simulink model "Ieee14_CC"  (R2023b)
settings: Solver=ode1  StartTime=0.0  StopTime=3600  FixedStep=1e-3  MaxStep=1e-4  RelTol=1e-3
model workspace (MAT data in the model file):
  pruebaValor = 0
libraries: dspnetwork x116, spsThreePhaseVIMeasurementLib x39, spsThreePhaseBreakerLib x21, spsLoadFlowBusLib x19, spsThreePhaseSeriesRLCBranchLib x16, spsThreePhaseFaultLib x16, source_mod x14, spsThreePhaseTransformerTwoWindingsLib x4, spsThreePhaseSourceLib x2, simulink x1, spspowerguiLib x1
(part 2 of 3)

== system Ieee14_CC/CB 0 ==
  Terminator : Terminator
  Three-Phase Breaker3 : spsThreePhaseBreakerLib/Three-Phase Breaker  InitialState=closed  SwitchA=on  SwitchB=on  SwitchC=on  SwitchTimes=[0.2]  External=on  BreakerResistance=0.01  SnubberResistance=1e6  SnubberCapacitance=inf  Measurements=Breaker voltages and currents
  UDP Receive : dspnetwork/UDP Receive  localURL='0.0.0.0'  localPort=30000  remoteURL='0.0.0.0'  remotePort=-1  recvBufferSize=2  dims=1  signalDatatype=uint16  isComplex=off  isVarSize=off  showBlockingTime=on  blockingTime=0  sampletime=0.1  blockPlatform=LINUX
  a : PMIOPort  Side=Left
  b : PMIOPort  Port=2  Side=Left
  c : PMIOPort  Port=3  Side=Left
  A : PMIOPort  Port=4  Side=Right
  B : PMIOPort  Port=5  Side=Right
  C : PMIOPort  Port=6  Side=Right
  com : Outport
  wires:
  UDP Receive/1 -> Three-Phase Breaker3/1, com/1
  UDP Receive/2 -> Terminator/1
  connections:
  b/RConn1 -- Three-Phase Breaker3/RConn2
  c/RConn1 -- Three-Phase Breaker3/RConn3
  A/RConn1 -- Three-Phase Breaker3/LConn1
  Three-Phase Breaker3/LConn2 -- B/RConn1
  C/RConn1 -- Three-Phase Breaker3/LConn3
  a/RConn1 -- Three-Phase Breaker3/RConn1

== system Ieee14_CC/CB 1 ==
  Terminator : Terminator
  Three-Phase Breaker3 : spsThreePhaseBreakerLib/Three-Phase Breaker  InitialState=closed  SwitchA=on  SwitchB=on  SwitchC=on  SwitchTimes=[0.2]  External=on  BreakerResistance=0.01  SnubberResistance=1e6  SnubberCapacitance=inf  Measurements=Breaker voltages and currents
  UDP Receive : dspnetwork/UDP Receive  localURL='0.0.0.0'  localPort=30001  remoteURL='0.0.0.0'  remotePort=-1  recvBufferSize=2  dims=1  signalDatatype=uint16  isComplex=off  isVarSize=off  showBlockingTime=on  blockingTime=0  sampletime=0.1  blockPlatform=LINUX
  a : PMIOPort  Side=Left
  b : PMIOPort  Port=2  Side=Left
  c : PMIOPort  Port=3  Side=Left
  A : PMIOPort  Port=4  Side=Right
  B : PMIOPort  Port=5  Side=Right
  C : PMIOPort  Port=6  Side=Right
  com : Outport
  wires:
  UDP Receive/1 -> Three-Phase Breaker3/1, com/1
  UDP Receive/2 -> Terminator/1
  connections:
  b/RConn1 -- Three-Phase Breaker3/RConn2
  c/RConn1 -- Three-Phase Breaker3/RConn3
  A/RConn1 -- Three-Phase Breaker3/LConn1
  Three-Phase Breaker3/LConn2 -- B/RConn1
  C/RConn1 -- Three-Phase Breaker3/LConn3
  a/RConn1 -- Three-Phase Breaker3/RConn1

== system Ieee14_CC/CB 10 ==
  Terminator : Terminator
  Three-Phase Breaker3 : spsThreePhaseBreakerLib/Three-Phase Breaker  InitialState=closed  SwitchA=on  SwitchB=on  SwitchC=on  SwitchTimes=[0.2]  External=on  BreakerResistance=0.01  SnubberResistance=1e6  SnubberCapacitance=inf  Measurements=Breaker voltages and currents
  UDP Receive : dspnetwork/UDP Receive  localURL='0.0.0.0'  localPort=30010  remoteURL='0.0.0.0'  remotePort=-1  recvBufferSize=2  dims=1  signalDatatype=uint16  isComplex=off  isVarSize=off  showBlockingTime=on  blockingTime=0  sampletime=0.1  blockPlatform=LINUX
  a : PMIOPort  Side=Left
  b : PMIOPort  Port=2  Side=Left
  c : PMIOPort  Port=3  Side=Left
  A : PMIOPort  Port=4  Side=Right
  B : PMIOPort  Port=5  Side=Right
  C : PMIOPort  Port=6  Side=Right
  com : Outport
  wires:
  UDP Receive/1 -> Three-Phase Breaker3/1, com/1
  UDP Receive/2 -> Terminator/1
  connections:
  b/RConn1 -- Three-Phase Breaker3/RConn2
  c/RConn1 -- Three-Phase Breaker3/RConn3
  A/RConn1 -- Three-Phase Breaker3/LConn1
  Three-Phase Breaker3/LConn2 -- B/RConn1
  C/RConn1 -- Three-Phase Breaker3/LConn3
  a/RConn1 -- Three-Phase Breaker3/RConn1

== system Ieee14_CC/CB 11 ==
  Terminator : Terminator
  Three-Phase Breaker3 : spsThreePhaseBreakerLib/Three-Phase Breaker  InitialState=closed  SwitchA=on  SwitchB=on  SwitchC=on  SwitchTimes=[0.2]  External=on  BreakerResistance=0.01  SnubberResistance=1e6  SnubberCapacitance=inf  Measurements=Breaker voltages and currents
  UDP Receive : dspnetwork/UDP Receive  localURL='0.0.0.0'  localPort=30011  remoteURL='0.0.0.0'  remotePort=-1  recvBufferSize=2  dims=1  signalDatatype=uint16  isComplex=off  isVarSize=off  showBlockingTime=on  blockingTime=0  sampletime=0.1  blockPlatform=LINUX
  a : PMIOPort  Side=Left
  b : PMIOPort  Port=2  Side=Left
  c : PMIOPort  Port=3  Side=Left
  A : PMIOPort  Port=4  Side=Right
  B : PMIOPort  Port=5  Side=Right
  C : PMIOPort  Port=6  Side=Right
  com : Outport
  wires:
  UDP Receive/1 -> Three-Phase Breaker3/1, com/1
  UDP Receive/2 -> Terminator/1
  connections:
  b/RConn1 -- Three-Phase Breaker3/RConn2
  c/RConn1 -- Three-Phase Breaker3/RConn3
  A/RConn1 -- Three-Phase Breaker3/LConn1
  Three-Phase Breaker3/LConn2 -- B/RConn1
  C/RConn1 -- Three-Phase Breaker3/LConn3
  a/RConn1 -- Three-Phase Breaker3/RConn1

== system Ieee14_CC/CB 12 ==
  Terminator : Terminator
  Three-Phase Breaker3 : spsThreePhaseBreakerLib/Three-Phase Breaker  InitialState=closed  SwitchA=on  SwitchB=on  SwitchC=on  SwitchTimes=[0.2]  External=on  BreakerResistance=0.01  SnubberResistance=1e6  SnubberCapacitance=inf  Measurements=Breaker voltages and currents
  UDP Receive : dspnetwork/UDP Receive  localURL='0.0.0.0'  localPort=30012  remoteURL='0.0.0.0'  remotePort=-1  recvBufferSize=2  dims=1  signalDatatype=uint16  isComplex=off  isVarSize=off  showBlockingTime=on  blockingTime=0  sampletime=0.1  blockPlatform=LINUX
  a : PMIOPort  Side=Left
  b : PMIOPort  Port=2  Side=Left
  c : PMIOPort  Port=3  Side=Left
  A : PMIOPort  Port=4  Side=Right
  B : PMIOPort  Port=5  Side=Right
  C : PMIOPort  Port=6  Side=Right
  com : Outport
  wires:
  UDP Receive/1 -> Three-Phase Breaker3/1, com/1
  UDP Receive/2 -> Terminator/1
  connections:
  b/RConn1 -- Three-Phase Breaker3/RConn2
  c/RConn1 -- Three-Phase Breaker3/RConn3
  A/RConn1 -- Three-Phase Breaker3/LConn1
  Three-Phase Breaker3/LConn2 -- B/RConn1
  C/RConn1 -- Three-Phase Breaker3/LConn3
  a/RConn1 -- Three-Phase Breaker3/RConn1

== system Ieee14_CC/CB 13 ==
  Terminator : Terminator
  Three-Phase Breaker3 : spsThreePhaseBreakerLib/Three-Phase Breaker  InitialState=closed  SwitchA=on  SwitchB=on  SwitchC=on  SwitchTimes=[0.2]  External=on  BreakerResistance=0.01  SnubberResistance=1e6  SnubberCapacitance=inf  Measurements=Breaker voltages and currents
  UDP Receive : dspnetwork/UDP Receive  localURL='0.0.0.0'  localPort=30013  remoteURL='0.0.0.0'  remotePort=-1  recvBufferSize=2  dims=1  signalDatatype=uint16  isComplex=off  isVarSize=off  showBlockingTime=on  blockingTime=0  sampletime=0.1  blockPlatform=LINUX
  a : PMIOPort  Side=Left
  b : PMIOPort  Port=2  Side=Left
  c : PMIOPort  Port=3  Side=Left
  A : PMIOPort  Port=4  Side=Right
  B : PMIOPort  Port=5  Side=Right
  C : PMIOPort  Port=6  Side=Right
  com : Outport
  wires:
  UDP Receive/1 -> Three-Phase Breaker3/1, com/1
  UDP Receive/2 -> Terminator/1
  connections:
  b/RConn1 -- Three-Phase Breaker3/RConn2
  c/RConn1 -- Three-Phase Breaker3/RConn3
  A/RConn1 -- Three-Phase Breaker3/LConn1
  Three-Phase Breaker3/LConn2 -- B/RConn1
  C/RConn1 -- Three-Phase Breaker3/LConn3
  a/RConn1 -- Three-Phase Breaker3/RConn1

== system Ieee14_CC/CB 14 ==
  Terminator : Terminator
  Three-Phase Breaker3 : spsThreePhaseBreakerLib/Three-Phase Breaker  InitialState=closed  SwitchA=on  SwitchB=on  SwitchC=on  SwitchTimes=[0.2]  External=on  BreakerResistance=0.01  SnubberResistance=1e6  SnubberCapacitance=inf  Measurements=Breaker voltages and currents
  UDP Receive : dspnetwork/UDP Receive  localURL='0.0.0.0'  localPort=30014  remoteURL='0.0.0.0'  remotePort=-1  recvBufferSize=2  dims=1  signalDatatype=uint16  isComplex=off  isVarSize=off  showBlockingTime=on  blockingTime=0  sampletime=0.1  blockPlatform=LINUX
  a : PMIOPort  Side=Left
  b : PMIOPort  Port=2  Side=Left
  c : PMIOPort  Port=3  Side=Left
  A : PMIOPort  Port=4  Side=Right
  B : PMIOPort  Port=5  Side=Right
  C : PMIOPort  Port=6  Side=Right
  com : Outport
  wires:
  UDP Receive/1 -> Three-Phase Breaker3/1, com/1
  UDP Receive/2 -> Terminator/1
  connections:
  b/RConn1 -- Three-Phase Breaker3/RConn2
  c/RConn1 -- Three-Phase Breaker3/RConn3
  A/RConn1 -- Three-Phase Breaker3/LConn1
  Three-Phase Breaker3/LConn2 -- B/RConn1
  C/RConn1 -- Three-Phase Breaker3/LConn3
  a/RConn1 -- Three-Phase Breaker3/RConn1

== system Ieee14_CC/CB 15 ==
  Terminator : Terminator
  Three-Phase Breaker3 : spsThreePhaseBreakerLib/Three-Phase Breaker  InitialState=closed  SwitchA=on  SwitchB=on  SwitchC=on  SwitchTimes=[0.2]  External=on  BreakerResistance=0.01  SnubberResistance=1e6  SnubberCapacitance=inf  Measurements=Breaker voltages and currents
  UDP Receive : dspnetwork/UDP Receive  localURL='0.0.0.0'  localPort=30015  remoteURL='0.0.0.0'  remotePort=-1  recvBufferSize=2  dims=1  signalDatatype=uint16  isComplex=off  isVarSize=off  showBlockingTime=on  blockingTime=0  sampletime=0.1  blockPlatform=LINUX
  a : PMIOPort  Side=Left
  b : PMIOPort  Port=2  Side=Left
  c : PMIOPort  Port=3  Side=Left
  A : PMIOPort  Port=4  Side=Right
  B : PMIOPort  Port=5  Side=Right
  C : PMIOPort  Port=6  Side=Right
  com : Outport
  wires:
  UDP Receive/1 -> Three-Phase Breaker3/1, com/1
  UDP Receive/2 -> Terminator/1
  connections:
  b/RConn1 -- Three-Phase Breaker3/RConn2
  c/RConn1 -- Three-Phase Breaker3/RConn3
  A/RConn1 -- Three-Phase Breaker3/LConn1
  Three-Phase Breaker3/LConn2 -- B/RConn1
  C/RConn1 -- Three-Phase Breaker3/LConn3
  a/RConn1 -- Three-Phase Breaker3/RConn1

== system Ieee14_CC/CB 2 ==
  Terminator : Terminator
  Three-Phase Breaker3 : spsThreePhaseBreakerLib/Three-Phase Breaker  InitialState=closed  SwitchA=on  SwitchB=on  SwitchC=on  SwitchTimes=[0.2]  External=on  BreakerResistance=0.01  SnubberResistance=1e6  SnubberCapacitance=inf  Measurements=Breaker voltages and currents
  UDP Receive : dspnetwork/UDP Receive  localURL='0.0.0.0'  localPort=30002  remoteURL='0.0.0.0'  remotePort=-1  recvBufferSize=2  dims=1  signalDatatype=uint16  isComplex=off  isVarSize=off  showBlockingTime=on  blockingTime=0  sampletime=0.1  blockPlatform=LINUX
  a : PMIOPort  Side=Left
  b : PMIOPort  Port=2  Side=Left
  c : PMIOPort  Port=3  Side=Left
  A : PMIOPort  Port=4  Side=Right
  B : PMIOPort  Port=5  Side=Right
  C : PMIOPort  Port=6  Side=Right
  com : Outport
  wires:
  UDP Receive/1 -> Three-Phase Breaker3/1, com/1
  UDP Receive/2 -> Terminator/1
  connections:
  b/RConn1 -- Three-Phase Breaker3/RConn2
  c/RConn1 -- Three-Phase Breaker3/RConn3
  A/RConn1 -- Three-Phase Breaker3/LConn1
  Three-Phase Breaker3/LConn2 -- B/RConn1
  C/RConn1 -- Three-Phase Breaker3/LConn3
  a/RConn1 -- Three-Phase Breaker3/RConn1

== system Ieee14_CC/CB 3 ==
  Terminator : Terminator
  Three-Phase Breaker3 : spsThreePhaseBreakerLib/Three-Phase Breaker  InitialState=closed  SwitchA=on  SwitchB=on  SwitchC=on  SwitchTimes=[0.2]  External=on  BreakerResistance=0.01  SnubberResistance=1e6  SnubberCapacitance=inf  Measurements=Breaker voltages and currents
  UDP Receive : dspnetwork/UDP Receive  localURL='0.0.0.0'  localPort=30003  remoteURL='0.0.0.0'  remotePort=-1  recvBufferSize=2  dims=1  signalDatatype=uint16  isComplex=off  isVarSize=off  showBlockingTime=on  blockingTime=0  sampletime=0.1  blockPlatform=LINUX
  a : PMIOPort  Side=Left
  b : PMIOPort  Port=2  Side=Left
  c : PMIOPort  Port=3  Side=Left
  A : PMIOPort  Port=4  Side=Right
  B : PMIOPort  Port=5  Side=Right
  C : PMIOPort  Port=6  Side=Right
  com : Outport
  wires:
  UDP Receive/1 -> Three-Phase Breaker3/1, com/1
  UDP Receive/2 -> Terminator/1
  connections:
  b/RConn1 -- Three-Phase Breaker3/RConn2
  c/RConn1 -- Three-Phase Breaker3/RConn3
  A/RConn1 -- Three-Phase Breaker3/LConn1
  Three-Phase Breaker3/LConn2 -- B/RConn1
  C/RConn1 -- Three-Phase Breaker3/LConn3
  a/RConn1 -- Three-Phase Breaker3/RConn1

== system Ieee14_CC/CB 4 ==
  Terminator : Terminator
  Three-Phase Breaker3 : spsThreePhaseBreakerLib/Three-Phase Breaker  InitialState=closed  SwitchA=on  SwitchB=on  SwitchC=on  SwitchTimes=[0.2]  External=on  BreakerResistance=0.01  SnubberResistance=1e6  SnubberCapacitance=inf  Measurements=Breaker voltages and currents
  UDP Receive : dspnetwork/UDP Receive  localURL='0.0.0.0'  localPort=30004  remoteURL='0.0.0.0'  remotePort=-1  recvBufferSize=2  dims=1  signalDatatype=uint16  isComplex=off  isVarSize=off  showBlockingTime=on  blockingTime=0  sampletime=0.1  blockPlatform=LINUX
  a : PMIOPort  Side=Left
  b : PMIOPort  Port=2  Side=Left
  c : PMIOPort  Port=3  Side=Left
  A : PMIOPort  Port=4  Side=Right
  B : PMIOPort  Port=5  Side=Right
  C : PMIOPort  Port=6  Side=Right
  com : Outport
  wires:
  UDP Receive/1 -> Three-Phase Breaker3/1, com/1
  UDP Receive/2 -> Terminator/1
  connections:
  b/RConn1 -- Three-Phase Breaker3/RConn2
  c/RConn1 -- Three-Phase Breaker3/RConn3
  A/RConn1 -- Three-Phase Breaker3/LConn1
  Three-Phase Breaker3/LConn2 -- B/RConn1
  C/RConn1 -- Three-Phase Breaker3/LConn3
  a/RConn1 -- Three-Phase Breaker3/RConn1

== system Ieee14_CC/CB 5 ==
  Terminator : Terminator
  Three-Phase Breaker3 : spsThreePhaseBreakerLib/Three-Phase Breaker  InitialState=closed  SwitchA=on  SwitchB=on  SwitchC=on  SwitchTimes=[0.2]  External=on  BreakerResistance=0.01  SnubberResistance=1e6  SnubberCapacitance=inf  Measurements=Breaker voltages and currents
  UDP Receive : dspnetwork/UDP Receive  localURL='0.0.0.0'  localPort=30005  remoteURL='0.0.0.0'  remotePort=-1  recvBufferSize=2  dims=1  signalDatatype=uint16  isComplex=off  isVarSize=off  showBlockingTime=on  blockingTime=0  sampletime=0.1  blockPlatform=LINUX
  a : PMIOPort  Side=Left
  b : PMIOPort  Port=2  Side=Left
  c : PMIOPort  Port=3  Side=Left
  A : PMIOPort  Port=4  Side=Right
  B : PMIOPort  Port=5  Side=Right
  C : PMIOPort  Port=6  Side=Right
  com : Outport
  wires:
  UDP Receive/1 -> Three-Phase Breaker3/1, com/1
  UDP Receive/2 -> Terminator/1
  connections:
  b/RConn1 -- Three-Phase Breaker3/RConn2
  c/RConn1 -- Three-Phase Breaker3/RConn3
  A/RConn1 -- Three-Phase Breaker3/LConn1
  Three-Phase Breaker3/LConn2 -- B/RConn1
  C/RConn1 -- Three-Phase Breaker3/LConn3
  a/RConn1 -- Three-Phase Breaker3/RConn1

== system Ieee14_CC/CB 6 ==
  Terminator : Terminator
  Three-Phase Breaker3 : spsThreePhaseBreakerLib/Three-Phase Breaker  InitialState=closed  SwitchA=on  SwitchB=on  SwitchC=on  SwitchTimes=[0.2]  External=on  BreakerResistance=0.01  SnubberResistance=1e6  SnubberCapacitance=inf  Measurements=Breaker voltages and currents
  UDP Receive : dspnetwork/UDP Receive  localURL='0.0.0.0'  localPort=30006  remoteURL='0.0.0.0'  remotePort=-1  recvBufferSize=2  dims=1  signalDatatype=uint16  isComplex=off  isVarSize=off  showBlockingTime=on  blockingTime=0  sampletime=0.1  blockPlatform=LINUX
  a : PMIOPort  Side=Left
  b : PMIOPort  Port=2  Side=Left
  c : PMIOPort  Port=3  Side=Left
  A : PMIOPort  Port=4  Side=Right
  B : PMIOPort  Port=5  Side=Right
  C : PMIOPort  Port=6  Side=Right
  com : Outport
  wires:
  UDP Receive/1 -> Three-Phase Breaker3/1, com/1
  UDP Receive/2 -> Terminator/1
  connections:
  b/RConn1 -- Three-Phase Breaker3/RConn2
  c/RConn1 -- Three-Phase Breaker3/RConn3
  A/RConn1 -- Three-Phase Breaker3/LConn1
  Three-Phase Breaker3/LConn2 -- B/RConn1
  C/RConn1 -- Three-Phase Breaker3/LConn3
  a/RConn1 -- Three-Phase Breaker3/RConn1

== system Ieee14_CC/CB 7 ==
  Terminator : Terminator
  Three-Phase Breaker3 : spsThreePhaseBreakerLib/Three-Phase Breaker  InitialState=closed  SwitchA=on  SwitchB=on  SwitchC=on  SwitchTimes=[0.2]  External=on  BreakerResistance=0.01  SnubberResistance=1e6  SnubberCapacitance=inf  Measurements=Breaker voltages and currents
  UDP Receive : dspnetwork/UDP Receive  localURL='0.0.0.0'  localPort=30007  remoteURL='0.0.0.0'  remotePort=-1  recvBufferSize=2  dims=1  signalDatatype=uint16  isComplex=off  isVarSize=off  showBlockingTime=on  blockingTime=0  sampletime=0.1  blockPlatform=LINUX
  a : PMIOPort  Side=Left
  b : PMIOPort  Port=2  Side=Left
  c : PMIOPort  Port=3  Side=Left
  A : PMIOPort  Port=4  Side=Right
  B : PMIOPort  Port=5  Side=Right
  C : PMIOPort  Port=6  Side=Right
  com : Outport
  wires:
  UDP Receive/2 -> Terminator/1
  UDP Receive/1 -> com/1, Three-Phase Breaker3/1
  connections:
  a/RConn1 -- Three-Phase Breaker3/RConn1
  C/RConn1 -- Three-Phase Breaker3/LConn3
  Three-Phase Breaker3/LConn2 -- B/RConn1
  A/RConn1 -- Three-Phase Breaker3/LConn1
  c/RConn1 -- Three-Phase Breaker3/RConn3
  b/RConn1 -- Three-Phase Breaker3/RConn2

== system Ieee14_CC/CB 8 ==
  Terminator : Terminator
  Three-Phase Breaker3 : spsThreePhaseBreakerLib/Three-Phase Breaker  InitialState=closed  SwitchA=on  SwitchB=on  SwitchC=on  SwitchTimes=[0.2]  External=on  BreakerResistance=0.01  SnubberResistance=1e6  SnubberCapacitance=inf  Measurements=Breaker voltages and currents
  UDP Receive : dspnetwork/UDP Receive  localURL='0.0.0.0'  localPort=30008  remoteURL='0.0.0.0'  remotePort=-1  recvBufferSize=2  dims=1  signalDatatype=uint16  isComplex=off  isVarSize=off  showBlockingTime=on  blockingTime=0  sampletime=0.1  blockPlatform=LINUX
  a : PMIOPort  Side=Left
  b : PMIOPort  Port=2  Side=Left
  c : PMIOPort  Port=3  Side=Left
  A : PMIOPort  Port=4  Side=Right
  B : PMIOPort  Port=5  Side=Right
  C : PMIOPort  Port=6  Side=Right
  com : Outport
  wires:
  UDP Receive/2 -> Terminator/1
  UDP Receive/1 -> com/1, Three-Phase Breaker3/1
  connections:
  a/RConn1 -- Three-Phase Breaker3/RConn1
  C/RConn1 -- Three-Phase Breaker3/LConn3
  Three-Phase Breaker3/LConn2 -- B/RConn1
  A/RConn1 -- Three-Phase Breaker3/LConn1
  c/RConn1 -- Three-Phase Breaker3/RConn3
  b/RConn1 -- Three-Phase Breaker3/RConn2

== system Ieee14_CC/CB 9 ==
  Terminator : Terminator
  Three-Phase Breaker3 : spsThreePhaseBreakerLib/Three-Phase Breaker  InitialState=closed  SwitchA=on  SwitchB=on  SwitchC=on  SwitchTimes=[0.2]  External=on  BreakerResistance=0.01  SnubberResistance=1e6  SnubberCapacitance=inf  Measurements=Breaker voltages and currents
  UDP Receive : dspnetwork/UDP Receive  localURL='0.0.0.0'  localPort=30009  remoteURL='0.0.0.0'  remotePort=-1  recvBufferSize=2  dims=1  signalDatatype=uint16  isComplex=off  isVarSize=off  showBlockingTime=on  blockingTime=0  sampletime=0.1  blockPlatform=LINUX
  a : PMIOPort  Side=Left
  b : PMIOPort  Port=2  Side=Left
  c : PMIOPort  Port=3  Side=Left
  A : PMIOPort  Port=4  Side=Right
  B : PMIOPort  Port=5  Side=Right
  C : PMIOPort  Port=6  Side=Right
  com : Outport
  wires:
  UDP Receive/1 -> Three-Phase Breaker3/1, com/1
  UDP Receive/2 -> Terminator/1
  connections:
  b/RConn1 -- Three-Phase Breaker3/RConn2
  c/RConn1 -- Three-Phase Breaker3/RConn3
  A/RConn1 -- Three-Phase Breaker3/LConn1
  Three-Phase Breaker3/LConn2 -- B/RConn1
  C/RConn1 -- Three-Phase Breaker3/LConn3
  a/RConn1 -- Three-Phase Breaker3/RConn1

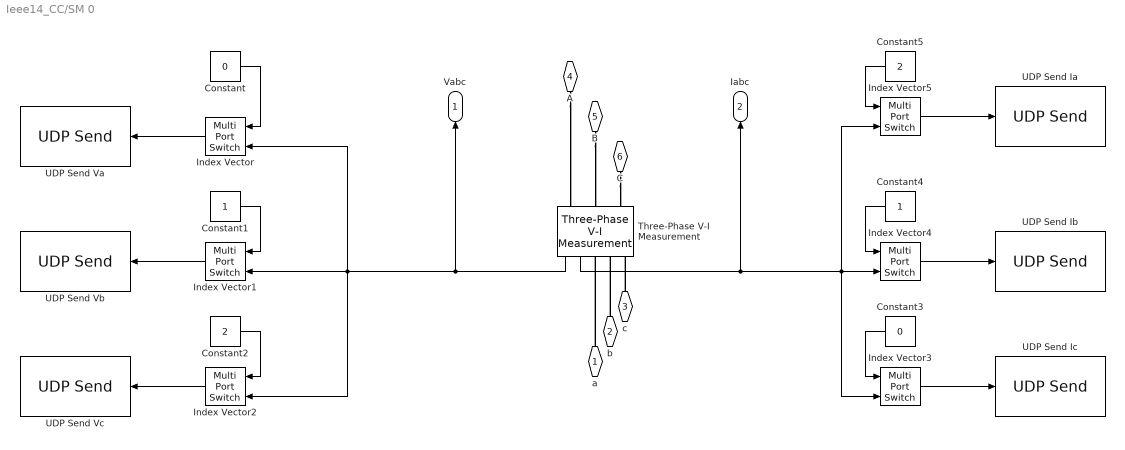
== system Ieee14_CC/SM 0 ==
  Constant : Constant  Value=0
  Constant1 : Constant
  Constant2 : Constant  Value=2
  Constant3 : Constant  Value=0
  Constant4 : Constant
  Constant5 : Constant  Value=2
  Index Vector{,1..5} (6 alike) : MultiPortSwitch  DataPortOrder=Zero-based contiguous  Inputs=1  zeroidx=on  SaturateOnIntegerOverflow=off  InputSameDT=off
  Three-Phase V-I Measurement : spsThreePhaseVIMeasurementLib/Three-Phase V-I Measurement  VoltageMeasurement=phase-to-ground  SetLabelV=off  LabelV=Vabc  Vpu=on  VpuLL=off  CurrentMeasurement=yes  SetLabelI=off  LabelI=Iabc  Ipu=on  Pbase=100e6  Vbase=69e3  OutputType=Complex  PhasorSimulation=off  PSBequivalent=0
  UDP Send Ia : dspnetwork/UDP Send  remoteURL='10.0.255.255'  remotePort=20002  localURL='255.255.255.255'  localPortSource=Automatically determine  localPort=-1  sendBufferSize=8192  sampletime=-1  blockPlatform=LINUX  separateLengthPort=0
  UDP Send Ib : dspnetwork/UDP Send  remoteURL='10.0.255.255'  remotePort=20001  localURL='255.255.255.255'  localPortSource=Automatically determine  localPort=-1  sendBufferSize=8192  sampletime=-1  blockPlatform=LINUX  separateLengthPort=0
  UDP Send Ic : dspnetwork/UDP Send  remoteURL='10.0.255.255'  remotePort=20000  localURL='255.255.255.255'  localPortSource=Automatically determine  localPort=-1  sendBufferSize=8192  sampletime=-1  blockPlatform=LINUX  separateLengthPort=0
  UDP Send Va : dspnetwork/UDP Send  remoteURL='10.0.255.255'  remotePort=10000  localURL='255.255.255.255'  localPortSource=Automatically determine  localPort=-1  sendBufferSize=8192  sampletime=-1  blockPlatform=LINUX  separateLengthPort=0
  UDP Send Vb : dspnetwork/UDP Send  remoteURL='10.0.255.255'  remotePort=10001  localURL='255.255.255.255'  localPortSource=Automatically determine  localPort=-1  sendBufferSize=8192  sampletime=-1  blockPlatform=LINUX  separateLengthPort=0
  UDP Send Vc : dspnetwork/UDP Send  remoteURL='10.0.255.255'  remotePort=10002  localURL='255.255.255.255'  localPortSource=Automatically determine  localPort=-1  sendBufferSize=8192  sampletime=-1  blockPlatform=LINUX  separateLengthPort=0
  a : PMIOPort  Side=Left
  b : PMIOPort  Port=2  Side=Left
  c : PMIOPort  Port=3  Side=Left
  A : PMIOPort  Port=4  Side=Right
  B : PMIOPort  Port=5  Side=Right
  C : PMIOPort  Port=6  Side=Right
  Vabc : Outport
  Iabc : Outport  Port=2
  wires:
  Index Vector/1 -> UDP Send Va/1
  Constant1/1 -> Index Vector1/1
  Constant/1 -> Index Vector/1
  Index Vector2/1 -> UDP Send Vc/1
  Index Vector1/1 -> UDP Send Vb/1
  Constant2/1 -> Index Vector2/1
  Three-Phase V-I Measurement/1 -> Index Vector2/2, Index Vector/2, Index Vector1/2, Vabc/1
  Index Vector4/1 -> UDP Send Ib/1
  Constant3/1 -> Index Vector3/1
  Index Vector3/1 -> UDP Send Ic/1
  Constant5/1 -> Index Vector5/1
  Constant4/1 -> Index Vector4/1
  Index Vector5/1 -> UDP Send Ia/1
  Three-Phase V-I Measurement/2 -> Iabc/1, Index Vector3/2, Index Vector4/2, Index Vector5/2
  connections:
  b/RConn1 -- Three-Phase V-I Measurement/RConn2
  a/RConn1 -- Three-Phase V-I Measurement/RConn1
  c/RConn1 -- Three-Phase V-I Measurement/RConn3
  A/RConn1 -- Three-Phase V-I Measurement/LConn1
  B/RConn1 -- Three-Phase V-I Measurement/LConn2
  C/RConn1 -- Three-Phase V-I Measurement/LConn3

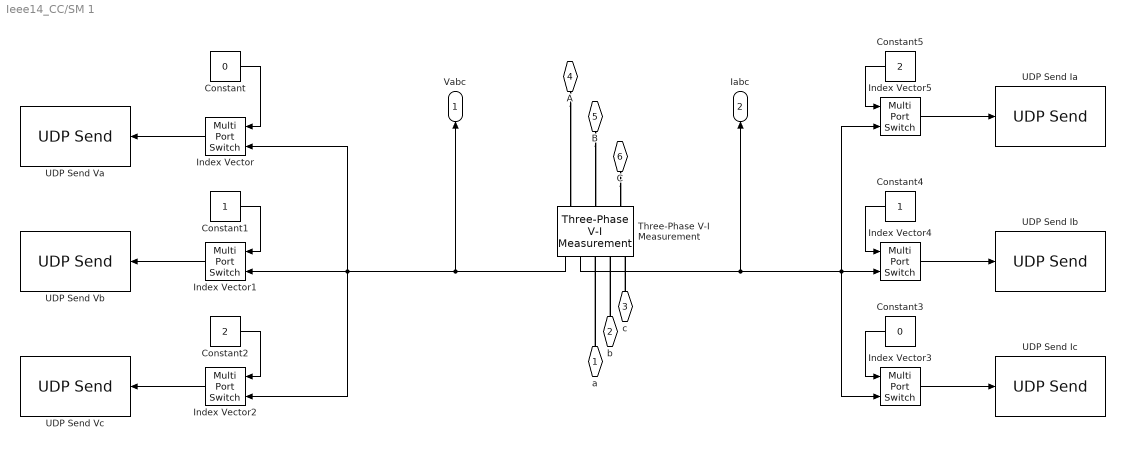
== system Ieee14_CC/SM 1 ==
  Constant : Constant  Value=0
  Constant1 : Constant
  Constant2 : Constant  Value=2
  Constant3 : Constant  Value=0
  Constant4 : Constant
  Constant5 : Constant  Value=2
  Index Vector{,1..5} (6 alike) : MultiPortSwitch  DataPortOrder=Zero-based contiguous  Inputs=1  zeroidx=on  SaturateOnIntegerOverflow=off  InputSameDT=off
  Three-Phase V-I Measurement : spsThreePhaseVIMeasurementLib/Three-Phase V-I Measurement  VoltageMeasurement=phase-to-ground  SetLabelV=off  LabelV=Vabc  Vpu=on  VpuLL=off  CurrentMeasurement=yes  SetLabelI=off  LabelI=Iabc  Ipu=on  Pbase=100e6  Vbase=69e3  OutputType=Complex  PhasorSimulation=off  PSBequivalent=0
  UDP Send Ia : dspnetwork/UDP Send  remoteURL='10.0.255.255'  remotePort=20012  localURL='255.255.255.255'  localPortSource=Automatically determine  localPort=-1  sendBufferSize=8192  sampletime=-1  blockPlatform=LINUX  separateLengthPort=0
  UDP Send Ib : dspnetwork/UDP Send  remoteURL='10.0.255.255'  remotePort=20011  localURL='255.255.255.255'  localPortSource=Automatically determine  localPort=-1  sendBufferSize=8192  sampletime=-1  blockPlatform=LINUX  separateLengthPort=0
  UDP Send Ic : dspnetwork/UDP Send  remoteURL='10.0.255.255'  remotePort=20010  localURL='255.255.255.255'  localPortSource=Automatically determine  localPort=-1  sendBufferSize=8192  sampletime=-1  blockPlatform=LINUX  separateLengthPort=0
  UDP Send Va : dspnetwork/UDP Send  remoteURL='10.0.255.255'  remotePort=10010  localURL='255.255.255.255'  localPortSource=Automatically determine  localPort=-1  sendBufferSize=8192  sampletime=-1  blockPlatform=LINUX  separateLengthPort=0
  UDP Send Vb : dspnetwork/UDP Send  remoteURL='10.0.255.255'  remotePort=10011  localURL='255.255.255.255'  localPortSource=Automatically determine  localPort=-1  sendBufferSize=8192  sampletime=-1  blockPlatform=LINUX  separateLengthPort=0
  UDP Send Vc : dspnetwork/UDP Send  remoteURL='10.0.255.255'  remotePort=10012  localURL='255.255.255.255'  localPortSource=Automatically determine  localPort=-1  sendBufferSize=8192  sampletime=-1  blockPlatform=LINUX  separateLengthPort=0
  a : PMIOPort  Side=Left
  b : PMIOPort  Port=2  Side=Left
  c : PMIOPort  Port=3  Side=Left
  A : PMIOPort  Port=4  Side=Right
  B : PMIOPort  Port=5  Side=Right
  C : PMIOPort  Port=6  Side=Right
  Vabc : Outport
  Iabc : Outport  Port=2
  wires:
  Index Vector/1 -> UDP Send Va/1
  Constant1/1 -> Index Vector1/1
  Constant/1 -> Index Vector/1
  Index Vector2/1 -> UDP Send Vc/1
  Index Vector1/1 -> UDP Send Vb/1
  Constant2/1 -> Index Vector2/1
  Three-Phase V-I Measurement/1 -> Index Vector2/2, Index Vector/2, Index Vector1/2, Vabc/1
  Index Vector4/1 -> UDP Send Ib/1
  Constant3/1 -> Index Vector3/1
  Index Vector3/1 -> UDP Send Ic/1
  Constant5/1 -> Index Vector5/1
  Constant4/1 -> Index Vector4/1
  Index Vector5/1 -> UDP Send Ia/1
  Three-Phase V-I Measurement/2 -> Iabc/1, Index Vector3/2, Index Vector4/2, Index Vector5/2
  connections:
  b/RConn1 -- Three-Phase V-I Measurement/RConn2
  a/RConn1 -- Three-Phase V-I Measurement/RConn1
  c/RConn1 -- Three-Phase V-I Measurement/RConn3
  A/RConn1 -- Three-Phase V-I Measurement/LConn1
  B/RConn1 -- Three-Phase V-I Measurement/LConn2
  C/RConn1 -- Three-Phase V-I Measurement/LConn3

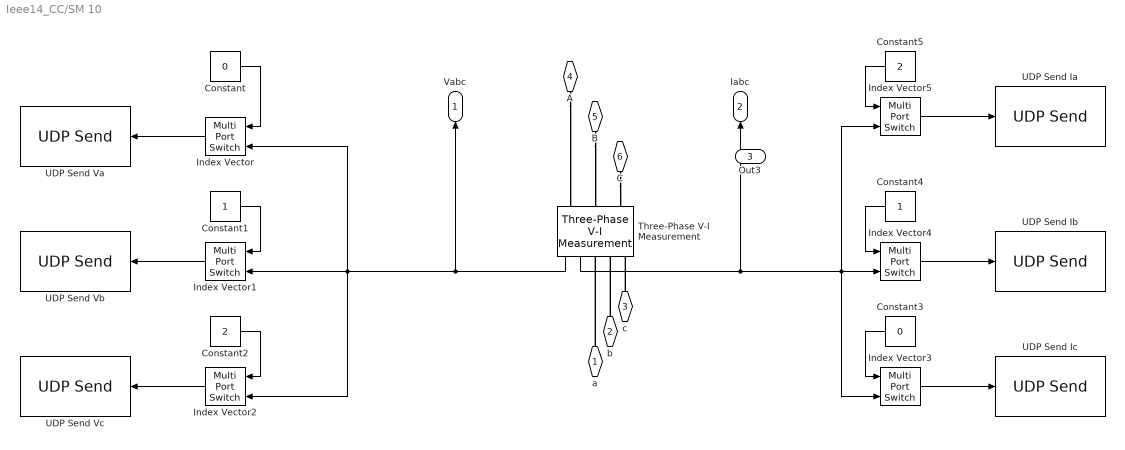
== system Ieee14_CC/SM 10 ==
  Constant : Constant  Value=0
  Constant1 : Constant
  Constant2 : Constant  Value=2
  Constant3 : Constant  Value=0
  Constant4 : Constant
  Constant5 : Constant  Value=2
  Index Vector{,1..5} (6 alike) : MultiPortSwitch  DataPortOrder=Zero-based contiguous  Inputs=1  zeroidx=on  SaturateOnIntegerOverflow=off  InputSameDT=off
  Three-Phase V-I Measurement : spsThreePhaseVIMeasurementLib/Three-Phase V-I Measurement  VoltageMeasurement=phase-to-ground  SetLabelV=off  LabelV=Vabc  Vpu=on  VpuLL=off  CurrentMeasurement=yes  SetLabelI=off  LabelI=Iabc  Ipu=on  Pbase=100e6  Vbase=69e3  OutputType=Complex  PhasorSimulation=off  PSBequivalent=0
  UDP Send Ia : dspnetwork/UDP Send  remoteURL='10.0.255.255'  remotePort=20102  localURL='255.255.255.255'  localPortSource=Automatically determine  localPort=-1  sendBufferSize=8192  sampletime=-1  blockPlatform=LINUX  separateLengthPort=0
  UDP Send Ib : dspnetwork/UDP Send  remoteURL='10.0.255.255'  remotePort=20101  localURL='255.255.255.255'  localPortSource=Automatically determine  localPort=-1  sendBufferSize=8192  sampletime=-1  blockPlatform=LINUX  separateLengthPort=0
  UDP Send Ic : dspnetwork/UDP Send  remoteURL='10.0.255.255'  remotePort=20100  localURL='255.255.255.255'  localPortSource=Automatically determine  localPort=-1  sendBufferSize=8192  sampletime=-1  blockPlatform=LINUX  separateLengthPort=0
  UDP Send Va : dspnetwork/UDP Send  remoteURL='10.0.255.255'  remotePort=10100  localURL='255.255.255.255'  localPortSource=Automatically determine  localPort=-1  sendBufferSize=8192  sampletime=-1  blockPlatform=LINUX  separateLengthPort=0
  UDP Send Vb : dspnetwork/UDP Send  remoteURL='10.0.255.255'  remotePort=10101  localURL='255.255.255.255'  localPortSource=Automatically determine  localPort=-1  sendBufferSize=8192  sampletime=-1  blockPlatform=LINUX  separateLengthPort=0
  UDP Send Vc : dspnetwork/UDP Send  remoteURL='10.0.255.255'  remotePort=10102  localURL='255.255.255.255'  localPortSource=Automatically determine  localPort=-1  sendBufferSize=8192  sampletime=-1  blockPlatform=LINUX  separateLengthPort=0
  a : PMIOPort  Side=Left
  b : PMIOPort  Port=2  Side=Left
  c : PMIOPort  Port=3  Side=Left
  A : PMIOPort  Port=4  Side=Right
  B : PMIOPort  Port=5  Side=Right
  C : PMIOPort  Port=6  Side=Right
  Vabc : Outport
  Iabc : Outport  Port=2
  Out3 : Outport  Port=3
  wires:
  Index Vector/1 -> UDP Send Va/1
  Constant1/1 -> Index Vector1/1
  Constant/1 -> Index Vector/1
  Index Vector2/1 -> UDP Send Vc/1
  Index Vector1/1 -> UDP Send Vb/1
  Constant2/1 -> Index Vector2/1
  Three-Phase V-I Measurement/1 -> Index Vector2/2, Index Vector/2, Index Vector1/2, Vabc/1
  Index Vector4/1 -> UDP Send Ib/1
  Constant3/1 -> Index Vector3/1
  Index Vector3/1 -> UDP Send Ic/1
  Constant5/1 -> Index Vector5/1
  Constant4/1 -> Index Vector4/1
  Index Vector5/1 -> UDP Send Ia/1
  Three-Phase V-I Measurement/2 -> Iabc/1, Index Vector3/2, Index Vector4/2, Index Vector5/2
  connections:
  b/RConn1 -- Three-Phase V-I Measurement/RConn2
  a/RConn1 -- Three-Phase V-I Measurement/RConn1
  c/RConn1 -- Three-Phase V-I Measurement/RConn3
  A/RConn1 -- Three-Phase V-I Measurement/LConn1
  B/RConn1 -- Three-Phase V-I Measurement/LConn2
  C/RConn1 -- Three-Phase V-I Measurement/LConn3

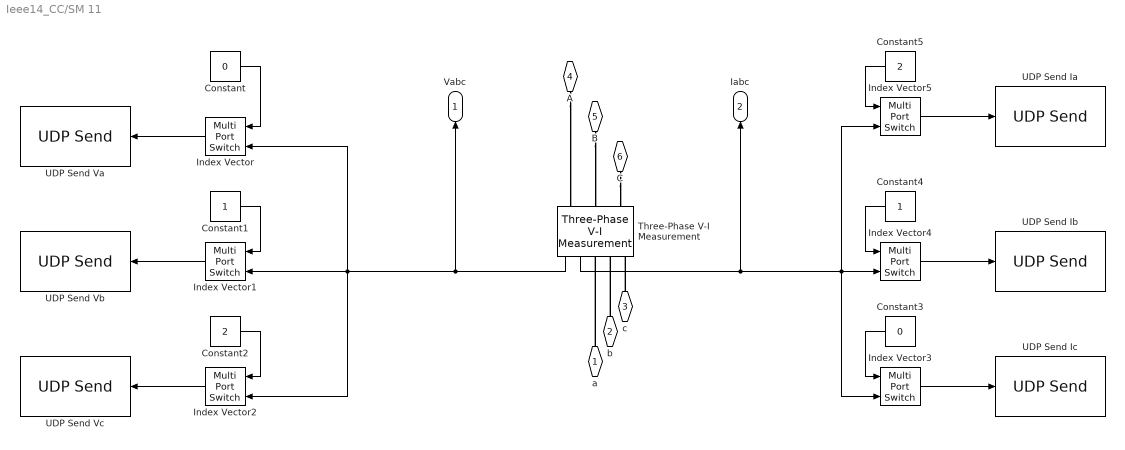
== system Ieee14_CC/SM 11 ==
  Constant : Constant  Value=0
  Constant1 : Constant
  Constant2 : Constant  Value=2
  Constant3 : Constant  Value=0
  Constant4 : Constant
  Constant5 : Constant  Value=2
  Index Vector{,1..5} (6 alike) : MultiPortSwitch  DataPortOrder=Zero-based contiguous  Inputs=1  zeroidx=on  SaturateOnIntegerOverflow=off  InputSameDT=off
  Three-Phase V-I Measurement : spsThreePhaseVIMeasurementLib/Three-Phase V-I Measurement  VoltageMeasurement=phase-to-ground  SetLabelV=off  LabelV=Vabc  Vpu=on  VpuLL=off  CurrentMeasurement=yes  SetLabelI=off  LabelI=Iabc  Ipu=on  Pbase=100e6  Vbase=69e3  OutputType=Complex  PhasorSimulation=off  PSBequivalent=0
  UDP Send Ia : dspnetwork/UDP Send  remoteURL='10.0.255.255'  remotePort=20112  localURL='255.255.255.255'  localPortSource=Automatically determine  localPort=-1  sendBufferSize=8192  sampletime=-1  blockPlatform=LINUX  separateLengthPort=0
  UDP Send Ib : dspnetwork/UDP Send  remoteURL='10.0.255.255'  remotePort=20111  localURL='255.255.255.255'  localPortSource=Automatically determine  localPort=-1  sendBufferSize=8192  sampletime=-1  blockPlatform=LINUX  separateLengthPort=0
  UDP Send Ic : dspnetwork/UDP Send  remoteURL='10.0.255.255'  remotePort=20110  localURL='255.255.255.255'  localPortSource=Automatically determine  localPort=-1  sendBufferSize=8192  sampletime=-1  blockPlatform=LINUX  separateLengthPort=0
  UDP Send Va : dspnetwork/UDP Send  remoteURL='10.0.255.255'  remotePort=10110  localURL='255.255.255.255'  localPortSource=Automatically determine  localPort=-1  sendBufferSize=8192  sampletime=-1  blockPlatform=LINUX  separateLengthPort=0
  UDP Send Vb : dspnetwork/UDP Send  remoteURL='10.0.255.255'  remotePort=10111  localURL='255.255.255.255'  localPortSource=Automatically determine  localPort=-1  sendBufferSize=8192  sampletime=-1  blockPlatform=LINUX  separateLengthPort=0
  UDP Send Vc : dspnetwork/UDP Send  remoteURL='10.0.255.255'  remotePort=10112  localURL='255.255.255.255'  localPortSource=Automatically determine  localPort=-1  sendBufferSize=8192  sampletime=-1  blockPlatform=LINUX  separateLengthPort=0
  a : PMIOPort  Side=Left
  b : PMIOPort  Port=2  Side=Left
  c : PMIOPort  Port=3  Side=Left
  A : PMIOPort  Port=4  Side=Right
  B : PMIOPort  Port=5  Side=Right
  C : PMIOPort  Port=6  Side=Right
  Vabc : Outport
  Iabc : Outport  Port=2
  wires:
  Index Vector/1 -> UDP Send Va/1
  Constant1/1 -> Index Vector1/1
  Constant/1 -> Index Vector/1
  Index Vector2/1 -> UDP Send Vc/1
  Index Vector1/1 -> UDP Send Vb/1
  Constant2/1 -> Index Vector2/1
  Three-Phase V-I Measurement/1 -> Index Vector2/2, Index Vector/2, Index Vector1/2, Vabc/1
  Index Vector4/1 -> UDP Send Ib/1
  Constant3/1 -> Index Vector3/1
  Index Vector3/1 -> UDP Send Ic/1
  Constant5/1 -> Index Vector5/1
  Constant4/1 -> Index Vector4/1
  Index Vector5/1 -> UDP Send Ia/1
  Three-Phase V-I Measurement/2 -> Iabc/1, Index Vector3/2, Index Vector4/2, Index Vector5/2
  connections:
  b/RConn1 -- Three-Phase V-I Measurement/RConn2
  a/RConn1 -- Three-Phase V-I Measurement/RConn1
  c/RConn1 -- Three-Phase V-I Measurement/RConn3
  A/RConn1 -- Three-Phase V-I Measurement/LConn1
  B/RConn1 -- Three-Phase V-I Measurement/LConn2
  C/RConn1 -- Three-Phase V-I Measurement/LConn3

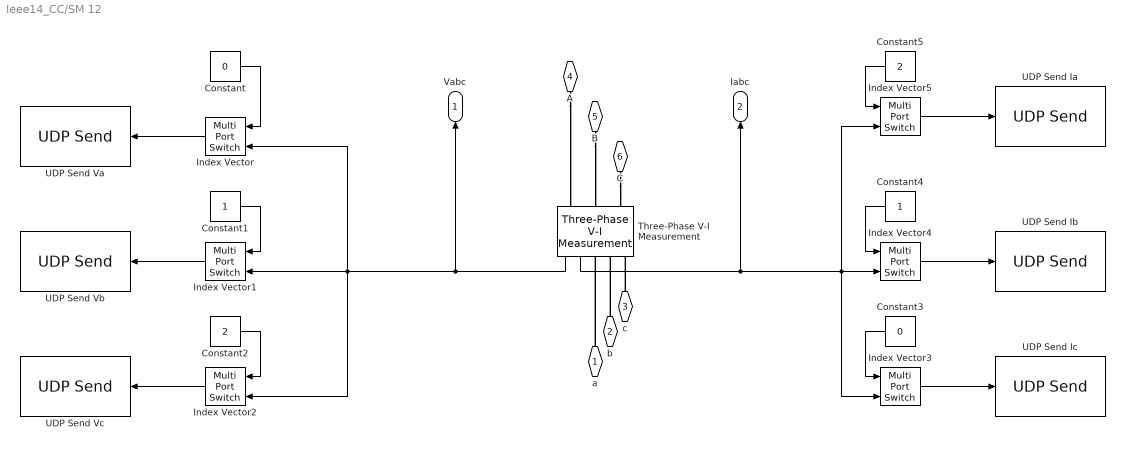
== system Ieee14_CC/SM 12 ==
  Constant : Constant  Value=0
  Constant1 : Constant
  Constant2 : Constant  Value=2
  Constant3 : Constant  Value=0
  Constant4 : Constant
  Constant5 : Constant  Value=2
  Index Vector{,1..5} (6 alike) : MultiPortSwitch  DataPortOrder=Zero-based contiguous  Inputs=1  zeroidx=on  SaturateOnIntegerOverflow=off  InputSameDT=off
  Three-Phase V-I Measurement : spsThreePhaseVIMeasurementLib/Three-Phase V-I Measurement  VoltageMeasurement=phase-to-ground  SetLabelV=off  LabelV=Vabc  Vpu=on  VpuLL=off  CurrentMeasurement=yes  SetLabelI=off  LabelI=Iabc  Ipu=on  Pbase=100e6  Vbase=69e3  OutputType=Complex  PhasorSimulation=off  PSBequivalent=0
  UDP Send Ia : dspnetwork/UDP Send  remoteURL='10.0.255.255'  remotePort=20122  localURL='255.255.255.255'  localPortSource=Automatically determine  localPort=-1  sendBufferSize=8192  sampletime=-1  blockPlatform=LINUX  separateLengthPort=0
  UDP Send Ib : dspnetwork/UDP Send  remoteURL='10.0.255.255'  remotePort=20121  localURL='255.255.255.255'  localPortSource=Automatically determine  localPort=-1  sendBufferSize=8192  sampletime=-1  blockPlatform=LINUX  separateLengthPort=0
  UDP Send Ic : dspnetwork/UDP Send  remoteURL='10.0.255.255'  remotePort=20120  localURL='255.255.255.255'  localPortSource=Automatically determine  localPort=-1  sendBufferSize=8192  sampletime=-1  blockPlatform=LINUX  separateLengthPort=0
  UDP Send Va : dspnetwork/UDP Send  remoteURL='10.0.255.255'  remotePort=10120  localURL='255.255.255.255'  localPortSource=Automatically determine  localPort=-1  sendBufferSize=8192  sampletime=-1  blockPlatform=LINUX  separateLengthPort=0
  UDP Send Vb : dspnetwork/UDP Send  remoteURL='10.0.255.255'  remotePort=10121  localURL='255.255.255.255'  localPortSource=Automatically determine  localPort=-1  sendBufferSize=8192  sampletime=-1  blockPlatform=LINUX  separateLengthPort=0
  UDP Send Vc : dspnetwork/UDP Send  remoteURL='10.0.255.255'  remotePort=10122  localURL='255.255.255.255'  localPortSource=Automatically determine  localPort=-1  sendBufferSize=8192  sampletime=-1  blockPlatform=LINUX  separateLengthPort=0
  a : PMIOPort  Side=Left
  b : PMIOPort  Port=2  Side=Left
  c : PMIOPort  Port=3  Side=Left
  A : PMIOPort  Port=4  Side=Right
  B : PMIOPort  Port=5  Side=Right
  C : PMIOPort  Port=6  Side=Right
  Vabc : Outport
  Iabc : Outport  Port=2
  wires:
  Index Vector/1 -> UDP Send Va/1
  Constant1/1 -> Index Vector1/1
  Constant/1 -> Index Vector/1
  Index Vector2/1 -> UDP Send Vc/1
  Index Vector1/1 -> UDP Send Vb/1
  Constant2/1 -> Index Vector2/1
  Three-Phase V-I Measurement/1 -> Index Vector2/2, Index Vector/2, Index Vector1/2, Vabc/1
  Index Vector4/1 -> UDP Send Ib/1
  Constant3/1 -> Index Vector3/1
  Index Vector3/1 -> UDP Send Ic/1
  Constant5/1 -> Index Vector5/1
  Constant4/1 -> Index Vector4/1
  Index Vector5/1 -> UDP Send Ia/1
  Three-Phase V-I Measurement/2 -> Iabc/1, Index Vector3/2, Index Vector4/2, Index Vector5/2
  connections:
  b/RConn1 -- Three-Phase V-I Measurement/RConn2
  a/RConn1 -- Three-Phase V-I Measurement/RConn1
  c/RConn1 -- Three-Phase V-I Measurement/RConn3
  A/RConn1 -- Three-Phase V-I Measurement/LConn1
  B/RConn1 -- Three-Phase V-I Measurement/LConn2
  C/RConn1 -- Three-Phase V-I Measurement/LConn3

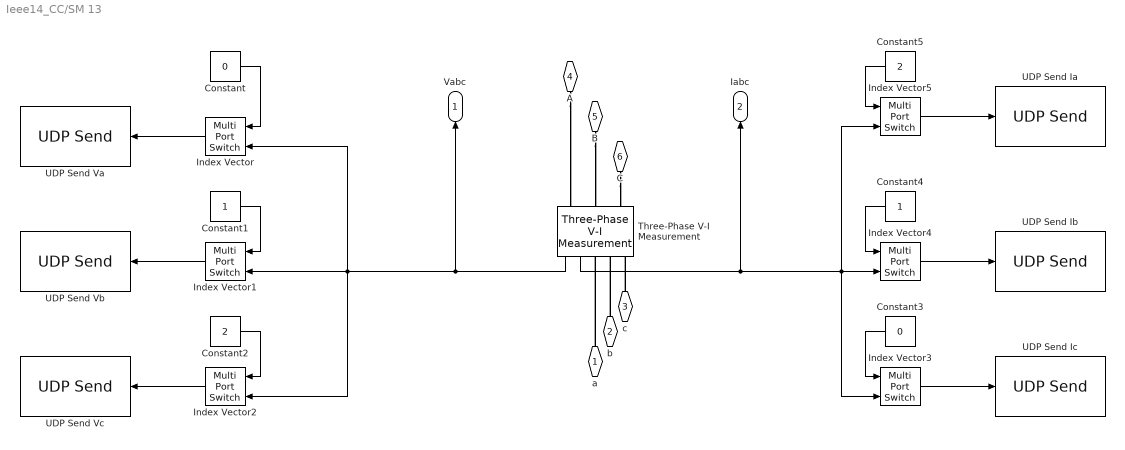
== system Ieee14_CC/SM 13 ==
  Constant : Constant  Value=0
  Constant1 : Constant
  Constant2 : Constant  Value=2
  Constant3 : Constant  Value=0
  Constant4 : Constant
  Constant5 : Constant  Value=2
  Index Vector{,1..5} (6 alike) : MultiPortSwitch  DataPortOrder=Zero-based contiguous  Inputs=1  zeroidx=on  SaturateOnIntegerOverflow=off  InputSameDT=off
  Three-Phase V-I Measurement : spsThreePhaseVIMeasurementLib/Three-Phase V-I Measurement  VoltageMeasurement=phase-to-ground  SetLabelV=off  LabelV=Vabc  Vpu=on  VpuLL=off  CurrentMeasurement=yes  SetLabelI=off  LabelI=Iabc  Ipu=on  Pbase=100e6  Vbase=69e3  OutputType=Complex  PhasorSimulation=off  PSBequivalent=0
  UDP Send Ia : dspnetwork/UDP Send  remoteURL='10.0.255.255'  remotePort=20132  localURL='255.255.255.255'  localPortSource=Automatically determine  localPort=-1  sendBufferSize=8192  sampletime=-1  blockPlatform=LINUX  separateLengthPort=0
  UDP Send Ib : dspnetwork/UDP Send  remoteURL='10.0.255.255'  remotePort=20131  localURL='255.255.255.255'  localPortSource=Automatically determine  localPort=-1  sendBufferSize=8192  sampletime=-1  blockPlatform=LINUX  separateLengthPort=0
  UDP Send Ic : dspnetwork/UDP Send  remoteURL='10.0.255.255'  remotePort=20130  localURL='255.255.255.255'  localPortSource=Automatically determine  localPort=-1  sendBufferSize=8192  sampletime=-1  blockPlatform=LINUX  separateLengthPort=0
  UDP Send Va : dspnetwork/UDP Send  remoteURL='10.0.255.255'  remotePort=10130  localURL='255.255.255.255'  localPortSource=Automatically determine  localPort=-1  sendBufferSize=8192  sampletime=-1  blockPlatform=LINUX  separateLengthPort=0
  UDP Send Vb : dspnetwork/UDP Send  remoteURL='10.0.255.255'  remotePort=10131  localURL='255.255.255.255'  localPortSource=Automatically determine  localPort=-1  sendBufferSize=8192  sampletime=-1  blockPlatform=LINUX  separateLengthPort=0
  UDP Send Vc : dspnetwork/UDP Send  remoteURL='10.0.255.255'  remotePort=10132  localURL='255.255.255.255'  localPortSource=Automatically determine  localPort=-1  sendBufferSize=8192  sampletime=-1  blockPlatform=LINUX  separateLengthPort=0
  a : PMIOPort  Side=Left
  b : PMIOPort  Port=2  Side=Left
  c : PMIOPort  Port=3  Side=Left
  A : PMIOPort  Port=4  Side=Right
  B : PMIOPort  Port=5  Side=Right
  C : PMIOPort  Port=6  Side=Right
  Vabc : Outport
  Iabc : Outport  Port=2
  wires:
  Index Vector/1 -> UDP Send Va/1
  Constant1/1 -> Index Vector1/1
  Constant/1 -> Index Vector/1
  Index Vector2/1 -> UDP Send Vc/1
  Index Vector1/1 -> UDP Send Vb/1
  Constant2/1 -> Index Vector2/1
  Three-Phase V-I Measurement/1 -> Index Vector2/2, Index Vector/2, Index Vector1/2, Vabc/1
  Index Vector4/1 -> UDP Send Ib/1
  Constant3/1 -> Index Vector3/1
  Index Vector3/1 -> UDP Send Ic/1
  Constant5/1 -> Index Vector5/1
  Constant4/1 -> Index Vector4/1
  Index Vector5/1 -> UDP Send Ia/1
  Three-Phase V-I Measurement/2 -> Iabc/1, Index Vector3/2, Index Vector4/2, Index Vector5/2
  connections:
  b/RConn1 -- Three-Phase V-I Measurement/RConn2
  a/RConn1 -- Three-Phase V-I Measurement/RConn1
  c/RConn1 -- Three-Phase V-I Measurement/RConn3
  A/RConn1 -- Three-Phase V-I Measurement/LConn1
  B/RConn1 -- Three-Phase V-I Measurement/LConn2
  C/RConn1 -- Three-Phase V-I Measurement/LConn3

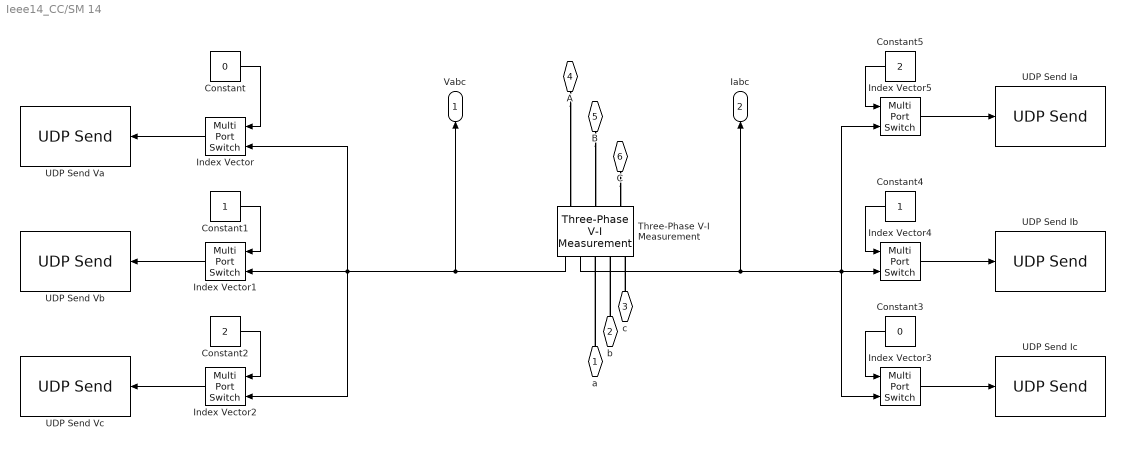
== system Ieee14_CC/SM 14 ==
  Constant : Constant  Value=0
  Constant1 : Constant
  Constant2 : Constant  Value=2
  Constant3 : Constant  Value=0
  Constant4 : Constant
  Constant5 : Constant  Value=2
  Index Vector{,1..5} (6 alike) : MultiPortSwitch  DataPortOrder=Zero-based contiguous  Inputs=1  zeroidx=on  SaturateOnIntegerOverflow=off  InputSameDT=off
  Three-Phase V-I Measurement : spsThreePhaseVIMeasurementLib/Three-Phase V-I Measurement  VoltageMeasurement=phase-to-ground  SetLabelV=off  LabelV=Vabc  Vpu=on  VpuLL=off  CurrentMeasurement=yes  SetLabelI=off  LabelI=Iabc  Ipu=on  Pbase=100e6  Vbase=69e3  OutputType=Complex  PhasorSimulation=off  PSBequivalent=0
  UDP Send Ia : dspnetwork/UDP Send  remoteURL='10.0.255.255'  remotePort=20142  localURL='255.255.255.255'  localPortSource=Automatically determine  localPort=-1  sendBufferSize=8192  sampletime=-1  blockPlatform=LINUX  separateLengthPort=0
  UDP Send Ib : dspnetwork/UDP Send  remoteURL='10.0.255.255'  remotePort=20141  localURL='255.255.255.255'  localPortSource=Automatically determine  localPort=-1  sendBufferSize=8192  sampletime=-1  blockPlatform=LINUX  separateLengthPort=0
  UDP Send Ic : dspnetwork/UDP Send  remoteURL='10.0.255.255'  remotePort=20140  localURL='255.255.255.255'  localPortSource=Automatically determine  localPort=-1  sendBufferSize=8192  sampletime=-1  blockPlatform=LINUX  separateLengthPort=0
  UDP Send Va : dspnetwork/UDP Send  remoteURL='10.0.255.255'  remotePort=10140  localURL='255.255.255.255'  localPortSource=Automatically determine  localPort=-1  sendBufferSize=8192  sampletime=-1  blockPlatform=LINUX  separateLengthPort=0
  UDP Send Vb : dspnetwork/UDP Send  remoteURL='10.0.255.255'  remotePort=10141  localURL='255.255.255.255'  localPortSource=Automatically determine  localPort=-1  sendBufferSize=8192  sampletime=-1  blockPlatform=LINUX  separateLengthPort=0
  UDP Send Vc : dspnetwork/UDP Send  remoteURL='10.0.255.255'  remotePort=10142  localURL='255.255.255.255'  localPortSource=Automatically determine  localPort=-1  sendBufferSize=8192  sampletime=-1  blockPlatform=LINUX  separateLengthPort=0
  a : PMIOPort  Side=Left
  b : PMIOPort  Port=2  Side=Left
  c : PMIOPort  Port=3  Side=Left
  A : PMIOPort  Port=4  Side=Right
  B : PMIOPort  Port=5  Side=Right
  C : PMIOPort  Port=6  Side=Right
  Vabc : Outport
  Iabc : Outport  Port=2
  wires:
  Index Vector/1 -> UDP Send Va/1
  Constant1/1 -> Index Vector1/1
  Constant/1 -> Index Vector/1
  Index Vector2/1 -> UDP Send Vc/1
  Index Vector1/1 -> UDP Send Vb/1
  Constant2/1 -> Index Vector2/1
  Three-Phase V-I Measurement/1 -> Index Vector2/2, Index Vector/2, Index Vector1/2, Vabc/1
  Index Vector4/1 -> UDP Send Ib/1
  Constant3/1 -> Index Vector3/1
  Index Vector3/1 -> UDP Send Ic/1
  Constant5/1 -> Index Vector5/1
  Constant4/1 -> Index Vector4/1
  Index Vector5/1 -> UDP Send Ia/1
  Three-Phase V-I Measurement/2 -> Iabc/1, Index Vector3/2, Index Vector4/2, Index Vector5/2
  connections:
  b/RConn1 -- Three-Phase V-I Measurement/RConn2
  a/RConn1 -- Three-Phase V-I Measurement/RConn1
  c/RConn1 -- Three-Phase V-I Measurement/RConn3
  A/RConn1 -- Three-Phase V-I Measurement/LConn1
  B/RConn1 -- Three-Phase V-I Measurement/LConn2
  C/RConn1 -- Three-Phase V-I Measurement/LConn3

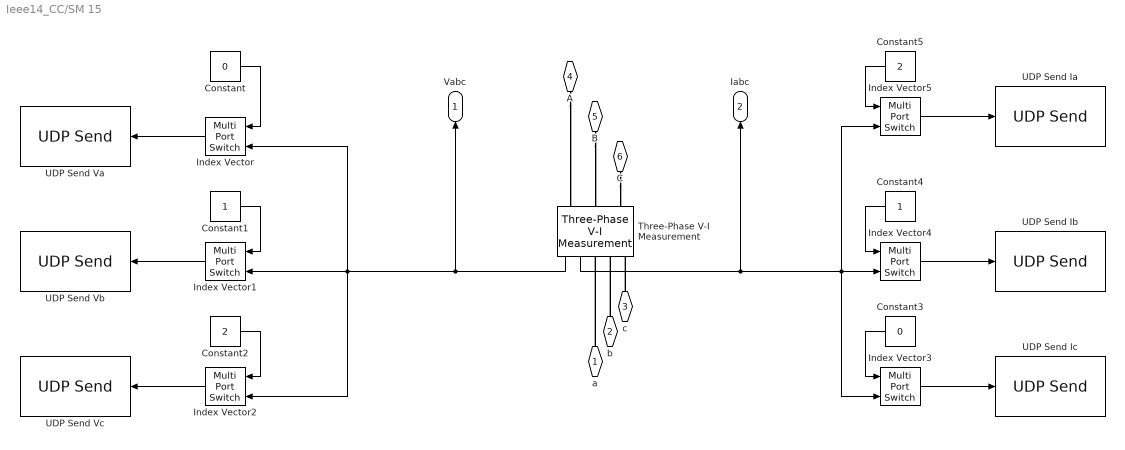
== system Ieee14_CC/SM 15 ==
  Constant : Constant  Value=0
  Constant1 : Constant
  Constant2 : Constant  Value=2
  Constant3 : Constant  Value=0
  Constant4 : Constant
  Constant5 : Constant  Value=2
  Index Vector{,1..5} (6 alike) : MultiPortSwitch  DataPortOrder=Zero-based contiguous  Inputs=1  zeroidx=on  SaturateOnIntegerOverflow=off  InputSameDT=off
  Three-Phase V-I Measurement : spsThreePhaseVIMeasurementLib/Three-Phase V-I Measurement  VoltageMeasurement=phase-to-ground  SetLabelV=off  LabelV=Vabc  Vpu=on  VpuLL=off  CurrentMeasurement=yes  SetLabelI=off  LabelI=Iabc  Ipu=on  Pbase=100e6  Vbase=69e3  OutputType=Complex  PhasorSimulation=off  PSBequivalent=0
  UDP Send Ia : dspnetwork/UDP Send  remoteURL='10.0.255.255'  remotePort=20152  localURL='255.255.255.255'  localPortSource=Automatically determine  localPort=-1  sendBufferSize=8192  sampletime=-1  blockPlatform=LINUX  separateLengthPort=0
  UDP Send Ib : dspnetwork/UDP Send  remoteURL='10.0.255.255'  remotePort=20151  localURL='255.255.255.255'  localPortSource=Automatically determine  localPort=-1  sendBufferSize=8192  sampletime=-1  blockPlatform=LINUX  separateLengthPort=0
  UDP Send Ic : dspnetwork/UDP Send  remoteURL='10.0.255.255'  remotePort=20150  localURL='255.255.255.255'  localPortSource=Automatically determine  localPort=-1  sendBufferSize=8192  sampletime=-1  blockPlatform=LINUX  separateLengthPort=0
  UDP Send Va : dspnetwork/UDP Send  remoteURL='10.0.255.255'  remotePort=10150  localURL='255.255.255.255'  localPortSource=Automatically determine  localPort=-1  sendBufferSize=8192  sampletime=-1  blockPlatform=LINUX  separateLengthPort=0
  UDP Send Vb : dspnetwork/UDP Send  remoteURL='10.0.255.255'  remotePort=10151  localURL='255.255.255.255'  localPortSource=Automatically determine  localPort=-1  sendBufferSize=8192  sampletime=-1  blockPlatform=LINUX  separateLengthPort=0
  UDP Send Vc : dspnetwork/UDP Send  remoteURL='10.0.255.255'  remotePort=10152  localURL='255.255.255.255'  localPortSource=Automatically determine  localPort=-1  sendBufferSize=8192  sampletime=-1  blockPlatform=LINUX  separateLengthPort=0
  a : PMIOPort  Side=Left
  b : PMIOPort  Port=2  Side=Left
  c : PMIOPort  Port=3  Side=Left
  A : PMIOPort  Port=4  Side=Right
  B : PMIOPort  Port=5  Side=Right
  C : PMIOPort  Port=6  Side=Right
  Vabc : Outport
  Iabc : Outport  Port=2
  wires:
  Index Vector/1 -> UDP Send Va/1
  Constant1/1 -> Index Vector1/1
  Constant/1 -> Index Vector/1
  Index Vector2/1 -> UDP Send Vc/1
  Index Vector1/1 -> UDP Send Vb/1
  Constant2/1 -> Index Vector2/1
  Three-Phase V-I Measurement/1 -> Index Vector2/2, Index Vector/2, Index Vector1/2, Vabc/1
  Index Vector4/1 -> UDP Send Ib/1
  Constant3/1 -> Index Vector3/1
  Index Vector3/1 -> UDP Send Ic/1
  Constant5/1 -> Index Vector5/1
  Constant4/1 -> Index Vector4/1
  Index Vector5/1 -> UDP Send Ia/1
  Three-Phase V-I Measurement/2 -> Iabc/1, Index Vector3/2, Index Vector4/2, Index Vector5/2
  connections:
  b/RConn1 -- Three-Phase V-I Measurement/RConn2
  a/RConn1 -- Three-Phase V-I Measurement/RConn1
  c/RConn1 -- Three-Phase V-I Measurement/RConn3
  A/RConn1 -- Three-Phase V-I Measurement/LConn1
  B/RConn1 -- Three-Phase V-I Measurement/LConn2
  C/RConn1 -- Three-Phase V-I Measurement/LConn3

== system Ieee14_CC/SM 2 ==
  Constant : Constant  Value=0
  Constant1 : Constant
  Constant2 : Constant  Value=2
  Constant3 : Constant  Value=0
  Constant4 : Constant
  Constant5 : Constant  Value=2
  Index Vector{,1..5} (6 alike) : MultiPortSwitch  DataPortOrder=Zero-based contiguous  Inputs=1  zeroidx=on  SaturateOnIntegerOverflow=off  InputSameDT=off
  Three-Phase V-I Measurement : spsThreePhaseVIMeasurementLib/Three-Phase V-I Measurement  VoltageMeasurement=phase-to-ground  SetLabelV=off  LabelV=Vabc  Vpu=on  VpuLL=off  CurrentMeasurement=yes  SetLabelI=off  LabelI=Iabc  Ipu=on  Pbase=100e6  Vbase=69e3  OutputType=Complex  PhasorSimulation=off  PSBequivalent=0
  UDP Send Ia : dspnetwork/UDP Send  remoteURL='10.0.255.255'  remotePort=20022  localURL='255.255.255.255'  localPortSource=Automatically determine  localPort=-1  sendBufferSize=8192  sampletime=-1  blockPlatform=LINUX  separateLengthPort=0
  UDP Send Ib : dspnetwork/UDP Send  remoteURL='10.0.255.255'  remotePort=20021  localURL='255.255.255.255'  localPortSource=Automatically determine  localPort=-1  sendBufferSize=8192  sampletime=-1  blockPlatform=LINUX  separateLengthPort=0
  UDP Send Ic : dspnetwork/UDP Send  remoteURL='10.0.255.255'  remotePort=20020  localURL='255.255.255.255'  localPortSource=Automatically determine  localPort=-1  sendBufferSize=8192  sampletime=-1  blockPlatform=LINUX  separateLengthPort=0
  UDP Send Va : dspnetwork/UDP Send  remoteURL='10.0.255.255'  remotePort=10020  localURL='255.255.255.255'  localPortSource=Automatically determine  localPort=-1  sendBufferSize=8192  sampletime=-1  blockPlatform=LINUX  separateLengthPort=0
  UDP Send Vb : dspnetwork/UDP Send  remoteURL='10.0.255.255'  remotePort=10021  localURL='255.255.255.255'  localPortSource=Automatically determine  localPort=-1  sendBufferSize=8192  sampletime=-1  blockPlatform=LINUX  separateLengthPort=0
  UDP Send Vc : dspnetwork/UDP Send  remoteURL='10.0.255.255'  remotePort=10022  localURL='255.255.255.255'  localPortSource=Automatically determine  localPort=-1  sendBufferSize=8192  sampletime=-1  blockPlatform=LINUX  separateLengthPort=0
  a : PMIOPort  Side=Left
  b : PMIOPort  Port=2  Side=Left
  c : PMIOPort  Port=3  Side=Left
  A : PMIOPort  Port=4  Side=Right
  B : PMIOPort  Port=5  Side=Right
  C : PMIOPort  Port=6  Side=Right
  Vabc : Outport
  Iabc : Outport  Port=2
  wires:
  Index Vector/1 -> UDP Send Va/1
  Constant1/1 -> Index Vector1/1
  Constant/1 -> Index Vector/1
  Index Vector2/1 -> UDP Send Vc/1
  Index Vector1/1 -> UDP Send Vb/1
  Constant2/1 -> Index Vector2/1
  Three-Phase V-I Measurement/1 -> Index Vector2/2, Index Vector/2, Index Vector1/2, Vabc/1
  Index Vector4/1 -> UDP Send Ib/1
  Constant3/1 -> Index Vector3/1
  Index Vector3/1 -> UDP Send Ic/1
  Constant5/1 -> Index Vector5/1
  Constant4/1 -> Index Vector4/1
  Index Vector5/1 -> UDP Send Ia/1
  Three-Phase V-I Measurement/2 -> Iabc/1, Index Vector3/2, Index Vector4/2, Index Vector5/2
  connections:
  b/RConn1 -- Three-Phase V-I Measurement/RConn2
  a/RConn1 -- Three-Phase V-I Measurement/RConn1
  c/RConn1 -- Three-Phase V-I Measurement/RConn3
  A/RConn1 -- Three-Phase V-I Measurement/LConn1
  B/RConn1 -- Three-Phase V-I Measurement/LConn2
  C/RConn1 -- Three-Phase V-I Measurement/LConn3
